simulink subsystem "rss_ModulElecAgCalcSenl"  (R2023a)
settings: Solver=VariableStepAuto  StartTime=0.0  StopTime=5  RelTol=1e-3
undefined symbols (not defined in the file): Cdbl_nElecAgSpdMaxVal, Cdbl_nElecAgSpdPeakVal, Cdbl_tiFstTaskSmpTi, ENM_MOTO_STATUS
libraries: lib_conversion x2, simulink x1, lib_discrete_time_integrator x1
settings Model: DefaultTestHarness=rss_electric_angle_compensation_thu  Creator=RAN2OFO  LastModifiedBy=xiaoqiang.yuan
settings OptimizationCC: ReuseModelBlockBuffer=off

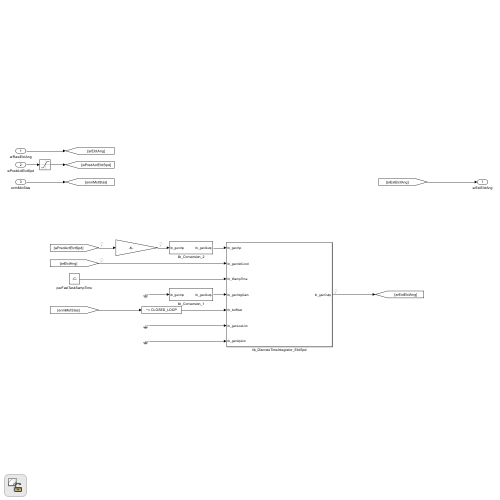
[thumbnail: Simulink's stored preview of the top-level diagram]
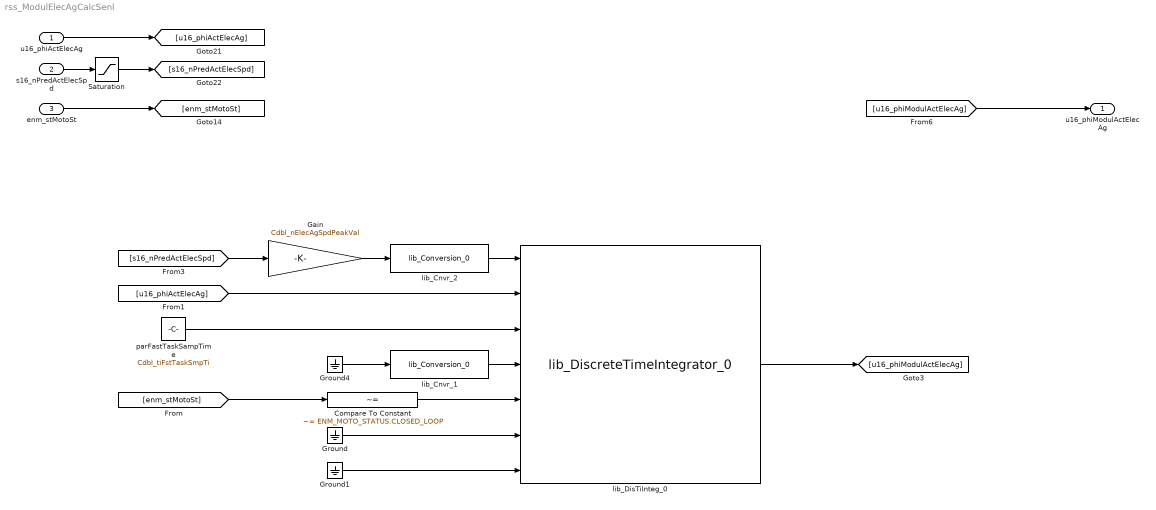
== system rss_ModulElecAgCalcSenl ==
  u16_phiActElecAg : Inport  OutDataTypeStr=dt_RadAng_u16r15b0
  s16_nPredActElecSpd : Inport  Port=2  OutDataTypeStr=dt_Standardize_s16p15b0
  enm_stMotoSt : Inport  Port=3  OutDataTypeStr=Enum: ENM_MOTO_STATUS  PortDimensions=1
  Compare To Constant : simulink/Logic and Bit Operations/Compare To Constant  relop=~=  const=ENM_MOTO_STATUS.CLOSED_LOOP  OutDataTypeStr=boolean
  Gain : Gain  Gain=Cdbl_nElecAgSpdPeakVal  OutDataTypeStr=Inherit: Inherit via back propagation
  Ground : Ground
  Ground1 : Ground
  Ground4 : Ground
  Saturation : Saturate  UpperLimit=Cdbl_nElecAgSpdMaxVal  LowerLimit=-Cdbl_nElecAgSpdMaxVal
  lib_Cnvr_1 : lib_conversion/lib_Conversion_0  lb_parDataType=uint8  lb_parOutpMaxVal=[]  lb_parOutpMinVal=[]  lb_parSatFlag=off
  lib_Cnvr_2 : lib_conversion/lib_Conversion_0  lb_parDataType=fixdt(1,16)  lb_parOutpMaxVal=Cdbl_nElecAgSpdPeakVal  lb_parOutpMinVal=[]  RndMeth=Simplest  lb_parSatFlag=off
  lib_DisTiInteg_0 : lib_discrete_time_integrator/lib_DiscreteTimeIntegrator_0  lb_parMaxInpVal=Cdbl_nElecAgSpdMaxVal*Cdbl_nElecAgSpdPeakVal  lb_parMinInpVal=-Cdbl_nElecAgSpdMaxVal*Cdbl_nElecAgSpdPeakVal  lb_parMaxSampTime=Cdbl_FstTaskSmpTiMaxVal  lb_parMaxIntgGain=0  lb_parAccmDataTypeMode=Same of output  lb_parOutpDataType=dt_RadAng_u16r15b0  lb_parIntgScopMode=Angular signal  lb_parSatFlag=off
  parFastTaskSampTime : Constant  Value=Cdbl_tiFstTaskSmpTi
  u16_phiModulActElecAg : Outport  OutDataTypeStr=dt_RadAng_u16r15b0
  wires:
  lib_Cnvr_1/1 -> lib_DisTiInteg_0/4
  [u16_phiModulActElecAg] -> u16_phiModulActElecAg/1
  Ground1/1 -> lib_DisTiInteg_0/7
  Ground/1 -> lib_DisTiInteg_0/6
  Ground4/1 -> lib_Cnvr_1/1
  parFastTaskSampTime/1 -> lib_DisTiInteg_0/3
  [u16_phiActElecAg] -> lib_DisTiInteg_0/2
  u16_phiActElecAg/1 -> [u16_phiActElecAg]
  s16_nPredActElecSpd/1 -> Saturation/1
  enm_stMotoSt/1 -> [enm_stMotoSt]
  [enm_stMotoSt] -> Compare To Constant/1
  Saturation/1 -> [s16_nPredActElecSpd]
  lib_DisTiInteg_0/1 -> [u16_phiModulActElecAg]
  Compare To Constant/1 -> lib_DisTiInteg_0/5
  [s16_nPredActElecSpd] -> Gain/1
  Gain/1 -> lib_Cnvr_2/1
  lib_Cnvr_2/1 -> lib_DisTiInteg_0/1
